simulink library "lib_AirProps_Viscosity"  (R2015a)
settings: Solver=ode45  StartTime=0.0  StopTime=10.0  RelTol=1e-3
settings Model: Creator=jlkratz  LastModifiedBy=jlkratz

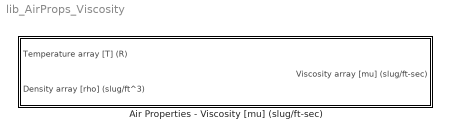
== system lib_AirProps_Viscosity ==
  Air Properties - Viscosity [mu] (slug/ft-sec) : Subsystem  mask(TSAT: Air Properties - Viscosity Block){BN_M=double(gcb)}
      mask prompts: BN_M "Block name"
      mask help:
      | This function provides an estimate of the viscosity of air given its temperature and denisty. The function uses empirical relations which are valid for dry air in the temperature range of 60K - 2000K (108R - 3600R) and pressures up to 2000MPa. See the block help menu for details. This function is capable of evaluating the viscosity for various temperature and density combinations at the same time given 1-D arrays of consistent lengths for both the temperature and density inputs.
      |
      | Units are clearly stated on the inport and outport so assure that your inputs are in the specified units and the output is properly converted to your desired units after the calculation.
      mask Help: web(which('AirProps_TSAT_Viscosity.html'),'-helpbrowser')

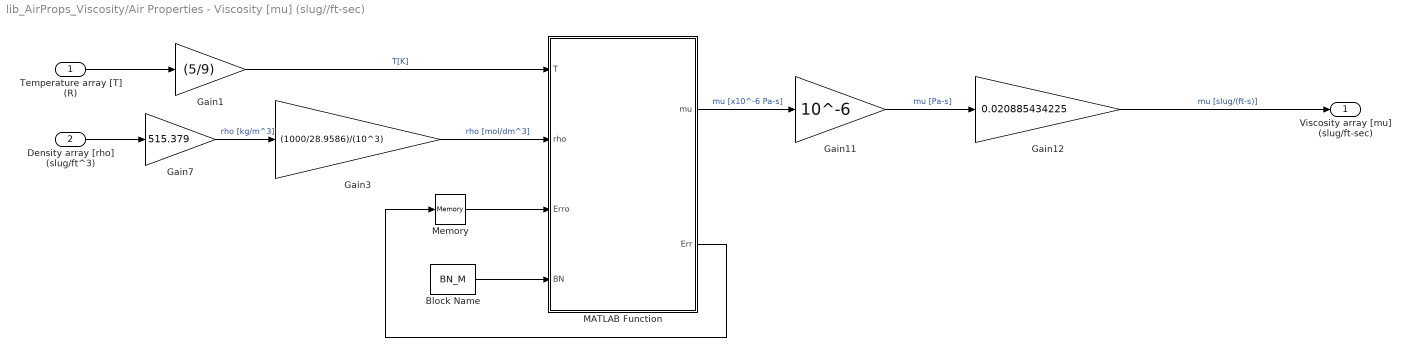
== system lib_AirProps_Viscosity/Air Properties - Viscosity [mu] (slug//ft-sec) ==
  Temperature array [T] (R) : Inport
  Density array [rho] (slug/ft^3) : Inport  Port=2
  Block Name : Constant  Value=BN_M
  Gain1 : Gain  Gain=(5/9)
  Gain11 : Gain  Gain=10^-6
  Gain12 : Gain  Gain=0.020885434225
  Gain3 : Gain  Gain=(1000/28.9586)/(10^3)
  Gain7 : Gain  Gain=515.379
  MATLAB Function : MATLAB Function  TreatAsAtomicUnit=on
  Memory : Memory  X0=zeros(1,3)
  Viscosity array [mu] (slug/ft-sec) : Outport
  wires:
  MATLAB Function/1(mu) -> Gain11/1  "mu [x10^-6 Pa-s]"
  Gain11/1 -> Gain12/1  "mu [Pa-s]"
  Gain12/1 -> Viscosity array [mu] (slug/ft-sec)/1  "mu [slug/(ft-s)]"
  Temperature array [T] (R)/1 -> Gain1/1
  Gain1/1 -> MATLAB Function/1(T)  "T[K]"
  Memory/1 -> MATLAB Function/3(Erro)
  MATLAB Function/2(Err) -> Memory/1
  Block Name/1 -> MATLAB Function/4(BN)
  Gain3/1 -> MATLAB Function/2(rho)  "rho [mol/dm^3]"
  Gain7/1 -> Gain3/1  "rho [kg/m^3]"
  Density array [rho] (slug/ft^3)/1 -> Gain7/1

== matlab function lib_AirProps_Viscosity/Air Properties - Viscosity [mu] (slug//ft-sec)/MATLAB Function ==
  data: T input; rho input; mu output; Erro input; BN input; Err output
function [mu,Err] = Viscosity_Air(T,rho,Erro,BN)
%#codegen

%Written By: Jonathan Kratz, NASA GRC
%Date: August 18, 2016
%Descirption: This function calculates the viscosity of air using
%empirical correlations from:
%   Lemmon, E., and Jacobsen, R., “Viscosity and Thermal Conductivity 
%   Equations for Nitrogen, Oxygen, Argon, and Air,” International Journal 
%   of Thermophysics, Vol. 25, No. 1, January 2004.
%
%Inputs:
%   T - Temperature array of the air in Kelvin (K)
%   rho - Density array of the air (mol/dm^3)
%
%Outputs:
%   mu - viscosity array corresponding to T (10x-6 Pa-sec)

%Number of element is T to solve for Cp
n = length(T);
m = length(rho);
mu = zeros(1,n);

%error checking
Err = Erro;
ErrNum = 1;
if n ~= m && Erro(ErrNum) == 0
    Err(ErrNum) = 1;
    fprintf('warning in %s: The input arrays T and rho must be the same length.\n',char(BN));
end
if min(T) < 60 && Erro(ErrNum) == 0
    Err(ErrNum) = 1;
    fprintf('warning in %s: At least 1 element of the temperature array is below the temperature range (60-2000K, 108-3600R) which the empirical correlation is valid\n',char(BN));
end
ErrNum = ErrNum + 1;
if max(T) > 2000 && Erro(ErrNum) == 0
    Err(ErrNum) = 1;
    fprintf('warning in %s: At least 1 element of the temperature array is above the temperature range (60-2000K, 108-3600R) which the empirical correlation is valid\n',char(BN));
end

%parameters%
Tc = 132.6312; %K
rhoc = 10.4477; %mol-dm^-3
M = 28.9586; %g/mol
eps_k = 103.3; %K
sig = 0.360; %nm

%Coefficients and exponents of the residual fluid viscosity equation
N = [10.72, 1.122, 0.002019, -8.876, -0.02916];
t = [0.2, 0.05, 2.4, 0.6, 3.6];
d = [1, 4, 9, 1, 8];
l = [0, 0, 0, 1, 1];

%Coefficients of the Collision Integral Equation
b = [0.431, -0.4623, 0.08406, 0.005341, -0.00331];

for j = 1:n
    %Calculate dilute gas viscosity
    Tstar = T(j)/eps_k;
    CIEsum = 0;
    for i = 1:5
        CIEsum = CIEsum + b(i)*log(Tstar)^(i-1);
    end
    OMEGA = exp(CIEsum);
    mu0 = (0.0266958*(M*T(j))^0.5)/(sig^2*OMEGA);
    %Calculate the residual gas viscosity
    mur = 0;
    gam = 0;
    for i = 1:5
        if l(i) == 0
            gam = 0;
        else
            gam = 1;
        end
        mur = mur + N(i)*(Tc/T(j))^t(i)*(rho(j)/rhoc)^d(i)*exp(-gam*(rho(j)/rhoc)^l(i));
    end
    %Calculate the overall viscosity
    mu(j) = mu0 + mur; %10^-6 Pa-s
end

end
